simulink model "task_8_model"  (R2020a)
settings: Solver=VariableStepAuto  StartTime=0.0  StopTime=10  RelTol=1e-3
values from neighbouring files (symbols this model uses):
  h = 1    [task_6.m]    (also in task_8.m; task_9.m)
  R = 1    [task_6.m]    (also in task_8.m; task_9.m)
  theta = data.theta.signals.values    [task_6.m]    (also in task_8.m = 0.523598775598)
undefined symbols (not defined in the file or in its folder): K
settings Model: Creator=jryl9  LastModifiedBy=jryl9

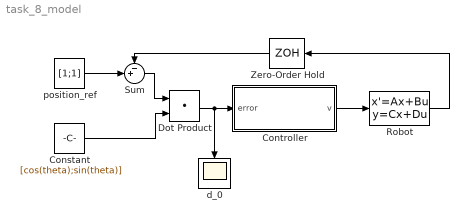
== system task_8_model ==
  Constant : Constant  Value=[cos(theta);sin(theta)]
  Controller : Subsystem
  Dot Product : DotProduct  InputSameDT=on  OutDataTypeStr=Inherit: Inherit via internal rule
  Robot : StateSpace  A=[0 0;0 0]  B=R*[cos(theta);sin(theta)]  C=[1 0;0 1]  D=[0; 0]  InitialCondition=0
  Sum : Sum  Inputs=-+|
  Zero-Order Hold : ZeroOrderHold  SampleTime=h
  d_0 : Scope
  position_ref : Constant  Value=[1;1]
  wires:
  Controller/1(v) -> Robot/1
  Robot/1 -> Zero-Order Hold/1
  Dot Product/1 -> d_0/1, Controller/1(error)
  position_ref/1 -> Sum/2
  Sum/1 -> Dot Product/1
  Constant/1 -> Dot Product/2
  Zero-Order Hold/1 -> Sum/1

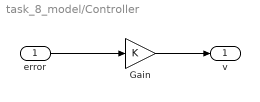
== system task_8_model/Controller ==
  error : Inport
  Gain : Gain  Gain=K
  v : Outport
  wires:
  Gain/1 -> v/1
  error/1 -> Gain/1
